simulink model "oneFingerSim"  (R2015b)
settings: Solver=VariableStepAuto  StartTime=0.0  StopTime=1.0  RelTol=1e-3
settings Model: Creator=Ricardo  LastModifiedBy=Ricardo

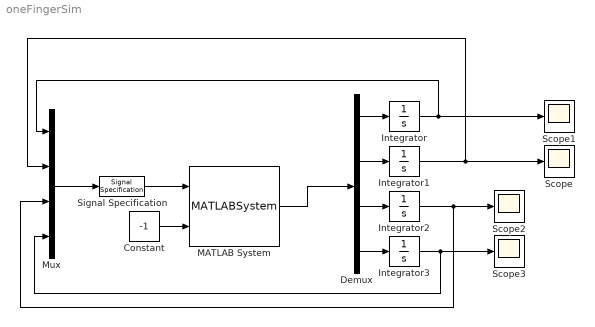
== system oneFingerSim ==
  Constant : Constant  Value=-1
  Demux : Demux
  Integrator : Integrator  InitialCondition=pi/10
  Integrator1 : Integrator  InitialCondition=pi/3
  Integrator2 : Integrator
  Integrator3 : Integrator
  MATLAB System : MATLABSystem  System=Finger  kP=1  kD=5  lP=0.1  lD=0.1  rP=0.02  rD=0.012  mP=0.02  mD=0.02  thetaP=pi/10  thetaD=pi/3  origin=[ 0, 0 ]  SimulateUsing=Interpreted execution
      mask Type: Finger
      mask Display:
      | disp('Finger');
      | port_label('input',1,'initVal');
      | port_label('input',2,'fa');
      | port_label('output',1,'xDot');
  Mux : Mux
  Scope{,1..3} (4 alike) : Scope
  Signal Specification : SignalSpecification  Dimensions=4
  wires:
  Demux/1 -> Integrator/1
  Demux/2 -> Integrator1/1
  Demux/3 -> Integrator2/1
  Demux/4 -> Integrator3/1
  Integrator1/1 -> Mux/2, Scope/1
  Integrator3/1 -> Mux/4, Scope3/1
  Integrator2/1 -> Mux/3, Scope2/1
  Mux/1 -> Signal Specification/1
  Signal Specification/1 -> MATLAB System/1
  MATLAB System/1 -> Demux/1
  Constant/1 -> MATLAB System/2
  Integrator/1 -> Mux/1, Scope1/1
